simulink model "Grafica2"  (R2019a)
settings: Solver=VariableStepAuto  StartTime=0.0  StopTime=20  RelTol=1e-3
settings Model: Creator=franc  LastModifiedBy=franc

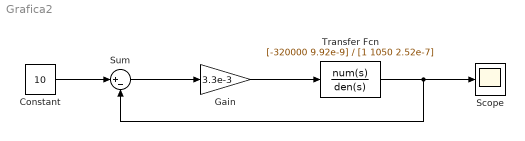
== system Grafica2 ==
  Constant : Constant  Value=10
  Gain : Gain  Gain=3.3e-3
  Scope : Scope
  Sum : Sum  Inputs=|+-
  Transfer Fcn : TransferFcn  Numerator=[-320000 9.92e-9]  Denominator=[1 1050 2.52e-7]
  wires:
  Constant/1 -> Sum/1
  Sum/1 -> Gain/1
  Gain/1 -> Transfer Fcn/1
  Transfer Fcn/1 -> Sum/2, Scope/1
